simulink model "useful_blocks"  (R2019a)
settings: Solver=VariableStepAuto  StartTime=0.0  StopTime=10.0  RelTol=1e-3
values from neighbouring files (symbols this model uses):
  I_CF_1_inv = inv(I_CF_1)    [set_params.m]
  M11 = [-b*k_f  b*k_f  b*k_f  -b*k_f ... (first row only)    [set_params.m]
  M2 = [  0       0      0       0 ... (first row only)    [set_params.m]
  omega_n = 50    [set_params.m]
  Ts = 0.01    [inner_pd_cs.m]    (also in set_params.m = 0.002)
  zeta = 0.55    [set_params.m]
libraries: simulink x1
settings Model: Creator=evgheniivolodscoi  LastModifiedBy=evgheniivolodscoi

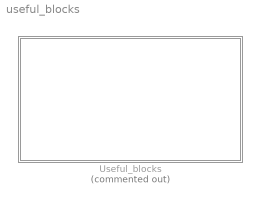
== system useful_blocks ==
  "Useful_blocks " : Subsystem  Commented=on

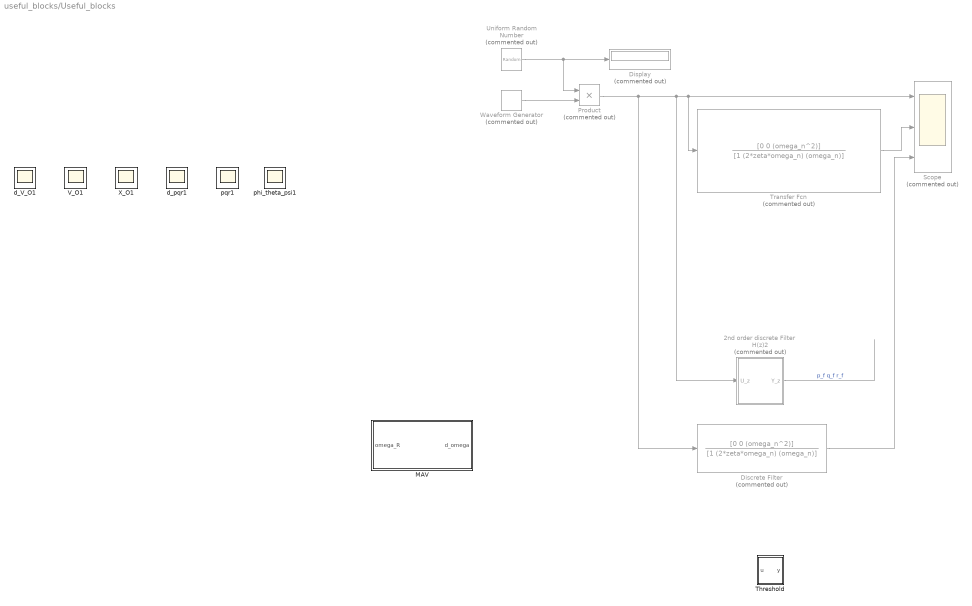
== system useful_blocks/Useful_blocks  ==
  2nd order discrete Filter H(z)2 : Subsystem  Commented=on
  Discrete Filter : DiscreteFilter  Commented=on  Numerator=[0 0 (omega_n^2)]  Denominator=[1 (2*zeta*omega_n) (omega_n)]
  Display : Display  Commented=on
  MAV : Subsystem
  Product : Product  Commented=on
  Scope : Scope  Commented=on  NumInputPorts=3
  Threshold : MATLAB Function  TreatAsAtomicUnit=on
  Transfer Fcn : TransferFcn  Commented=on  Numerator=[0 0 (omega_n^2)]  Denominator=[1 (2*zeta*omega_n) (omega_n)]
  Uniform Random Number : UniformRandomNumber  Commented=on  SampleTime=0.1
  V_O1 : Scope
  Waveform Generator : simulink/Sources/Waveform Generator  Commented=on  OutMin=[]  OutMax=[]  OutDataTypeStr=double  SelectedSignal=1  Signals=sin('Amplitude', 2, 'Frequency', 5, 'Phase', 0)  BlockNames=MultiportSwitch_c57f81d41abc4d6  SampleTime=0.1
      settings: SourceProductName=Simulink
  X_O1 : Scope
  d_V_O1 : Scope
  d_pqr1 : Scope
  phi_theta_psi1 : Scope
  pqr1 : Scope
  wires:
  ? -> pqr1/1
  ? -> d_V_O1/1
  ? -> V_O1/1
  ? -> phi_theta_psi1/1
  ? -> X_O1/1
  ? -> d_pqr1/1
  Product/1 -> Discrete Filter/1, 2nd order discrete Filter H(z)2/1(U_z), Transfer Fcn/1, Scope/1
  Discrete Filter/1 -> Scope/3
  2nd order discrete Filter H(z)2/1(Y_z) -> ?  "p_f q_f r_f"
  Waveform Generator/1 -> Product/2
  Transfer Fcn/1 -> Scope/2
  Uniform Random Number/1 -> Product/1, Display/1

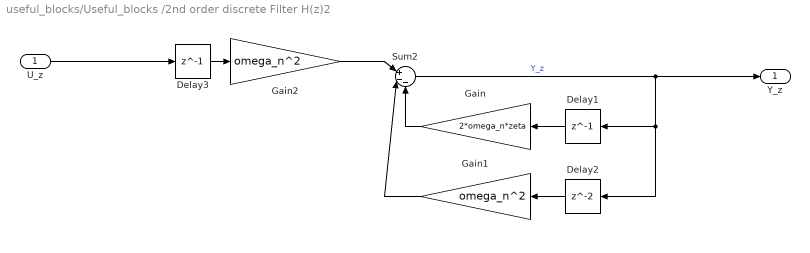
== system useful_blocks/Useful_blocks /2nd order discrete Filter H(z)2 ==
  U_z : Inport
  Delay1 : Delay  DelayLength=1  InitialCondition=0
  Delay2 : Delay  InitialCondition=0
  Delay3 : Delay  DelayLength=1  InitialCondition=0
  Gain : Gain  Gain=2*omega_n*zeta
  Gain1 : Gain  Gain=omega_n^2
  Gain2 : Gain  Gain=omega_n^2
  Sum2 : Sum  Inputs=|+--
  Y_z : Outport
  wires:
  Gain/1 -> Sum2/3
  U_z/1 -> Delay3/1
  Delay1/1 -> Gain/1
  Delay2/1 -> Gain1/1
  Gain1/1 -> Sum2/2
  Delay3/1 -> Gain2/1
  Gain2/1 -> Sum2/1
  Sum2/1 -> Y_z/1, Delay1/1, Delay2/1  "Y_z"

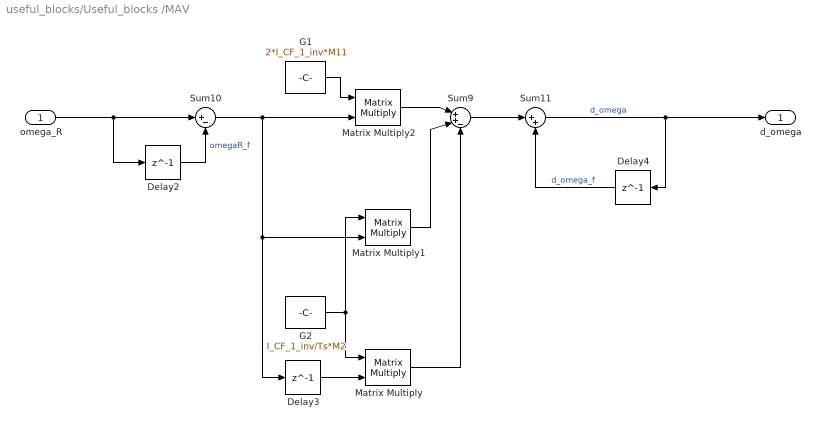
== system useful_blocks/Useful_blocks /MAV ==
  omega_R : Inport
  Delay2 : Delay  DelayLength=1
  Delay3 : Delay  DelayLength=1
  Delay4 : Delay  DelayLength=1
  G1 : Constant  Value=2*I_CF_1_inv*M11
  G2 : Constant  Value=I_CF_1_inv/Ts*M2
  Matrix Multiply : Product  Multiplication=Matrix(*)
  Matrix Multiply1 : Product  Multiplication=Matrix(*)
  Matrix Multiply2 : Product  Multiplication=Matrix(*)
  Sum10 : Sum  Inputs=|+-
  Sum11 : Sum  Inputs=|++
  Sum9 : Sum  Inputs=|++-
  d_omega : Outport
  wires:
  Matrix Multiply/1 -> Sum9/3
  Delay4/1 -> Sum11/2  "d_omega_f"
  Delay2/1 -> Sum10/2  "omegaR_f"
  Delay3/1 -> Matrix Multiply/2
  omega_R/1 -> Delay2/1, Sum10/1
  Sum9/1 -> Sum11/1
  Sum11/1 -> d_omega/1, Delay4/1  "d_omega"
  Sum10/1 -> Delay3/1, Matrix Multiply1/2, Matrix Multiply2/2
  Matrix Multiply2/1 -> Sum9/1
  Matrix Multiply1/1 -> Sum9/2
  G2/1 -> Matrix Multiply1/1, Matrix Multiply/1
  G1/1 -> Matrix Multiply2/1

== matlab function useful_blocks/Useful_blocks /Threshold ==
  data: u input; y output
function y = fcn(u)

for i=1:size(u, 1)
   if u(i) > 525
       u(i) = 525
   elseif u(i) < -525
       u(i) = -525
   end
end

y = u;
